simulink model "ansiBPF"  (R2018a)
settings: Solver=VariableStepAuto  StartTime=0.0  StopTime=0.001  RelTol=1e-3
undefined symbols (not defined in the file): fdesignblkfcn, G1, G10, G11, G12, G13, G14, G15, G16, G17, G18, G19, G2, G20, G21, G22, G23, G24, G25, G26, G3, G4, G5, G6, G7, G8, G9, gcbh, get, T
libraries: dspsrcs4 x1, dspxfrm3 x1, dspobslib x1
(part 8 of 8)

== system ansiBPF/Filter Bank /Filter 7/Bandpass Filter ==
  In : Inport
  Generated Filter Block : DiscreteFir  Tag=BlockMethodSubSystem  Coefficients=[-0.00513428504174898853 -0.000361211182980185862 -0.000373103186357564155 -0.000384811331785065228 -0.000396112667542441576 -0.000407118555369722311 -0.000417653688197336121 -0.000427763725028186906 -0.000437267124181367581 -0.000446249305343924966 -0.000454509424433863511 -0.000462144016945200342 -0.000468961541006500285 -0.00047510108603985809 -0.000480378661032834482 -0.000484955245458708502 -0.000488642490353076247 -0.000491641885964510974 -0.000493768806337300647 -0.000495248235932606025 -0.000495834603735094046 -0.000495723671978558081 -0.000494559737024913965 -0.000492503002177277277 -0.000489046555423059792 -0.000484334433113684567 -0.000477752667274562498 -0.000469736939490140309 -0.000459918134660938348 -0.000449820271314354311 -0.000440410655265032196 -0.000437343681880778001 -0.000415017077466513619 -0.000403028957904219749 -0.000387890543032657796 -0.000370831057829995689 -0.000352862955276029514 -0.000333297903416547386 -0.000312652166365081177 -0.000290495949674185797 -0.000267228447718805549 -0.000242500256187110872 -0.000216622507784609391 -0.000189306018353237692 -0.000160822312630247454 -0.00013090431231813814 -9.977491882814921e-05 -6.71828741737578035e-05 -3.3362190465583284e-05 1.87737953330797842e-06 3.82578750794589309e-05 7.59296875815955528e-05 0.000114590062210208948 0.000154392763453061534 0.000195060270031960137 0.000236865934738083922 0.000279648893625907338 0.000323829091085882251 0.000369138505596120121 0.000415800723553011854 0.000462889030708697757 0.000510071506735421164 0.000556666261009906545 0.000608453913411027272 0.000657171616570307086 0.000707564922296681671 0.000758656123872777834 0.000809979435514389368 0.000861877681813531566 0.000914029787083755823 0.000966573126424342326 0.00101924401116606795 0.00107213769902803134 0.00112502250686530997 0.00117793740491828791 0.00123065410311573283 0.00128320856734487278 0.00133542131582664548 0.00138735182905208717 0.00143883522759182827 0.00148991568918932895 0.00154040519539005148 0.00159031610175726043 0.00163940693647644841 0.00168764727947417928 0.00173477135550877495 0.00178082983361215483 0.00182567127317073566 0.0018695019177895505 0.00191212963348372819 0.00195362536784609393 0.00199334896058852478 0.00203113833753347474 0.00206700493227391681 0.0021029201432464506 0.00213512724940612131 0.00216618711059341461 0.00219526175881140173 0.0022220427721179898 0.00224678560238826585 0.00226918834154568681 0.00228934830816726479 0.00230704121418263746 0.00232235771406847031 0.00233510070426523435 0.00234530486231102541 0.00235276167382800173 0.00235749633401698133 0.00235933903264844667 0.00235834137161671951 0.00235436391360369047 0.00234747670652394984 0.00233755877697023988 0.00232468177547491897 0.00230868814289701641 0.00228959846568288668 0.00226721357335321659 0.00224160611906860582 0.00221267617648638086 0.00218063539614888561 0.00214536781771183446 0.00210698698475577035 0.00206506784763389392 0.00201966991007280225 0.00197100617659200792 0.00191989706014282762 0.00186440389211500507 0.00180628021157354097 0.00174486314747820904 0.00168008694999815535 0.00161223713228134309 0.00154115078309086367 0.00146698945678845746 0.00138969143960892649 0.00130944179231868717 0.0012262142007846452 0.00114015129668698623 0.00105121700108983256 0.000959543531271865027 0.00086511792793485579 0.000768083684632907249 0.000668448112385646451 0.000566380537741520483 0.000461926118994698733 0.000355279617939186323 0.000246467302056672586 0.000135638513742188267 2.27743015301716597e-05 -9.19400378440655725e-05 -0.000208443181019318563 -0.00032643762964840433 -0.000445883130048132853 -0.000566569052997391797 -0.000688684043530423361 -0.000811979045388096601 -0.000936108974577499705 -0.00106067060247101242 -0.00118658653091919348 -0.00131250527363708049 -0.00143887628290320321 -0.00156555167828120799 -0.00169215833900483942 -0.00181874382778180388 -0.0019450460938826577 -0.00207100845483666361 -0.00219634459459971607 -0.00232096893781466715 ...(+10100 chars)]  InputProcessing=Columns as channels (frame based)
  Out : Outport
  wires:
  In/1 -> Generated Filter Block/1
  Generated Filter Block/1 -> Out/1

== system ansiBPF/Filter Bank /Filter 8/Bandpass Filter ==
  In : Inport
  Generated Filter Block : DiscreteFir  Tag=BlockMethodSubSystem  Coefficients=[-0.00516622582828563971 -0.000470469850453975741 -0.000490549882434943539 -0.000510272576474730781 -0.000529259103219038157 -0.000547443950766350086 -0.000564418046489216681 -0.00058024415585958191 -0.000594695099131715976 -0.000608171258508255833 -0.000620765185585862335 -0.000633135229341045234 -0.000645123384864209996 -0.000656270670386141161 -0.000663245745322524859 -0.000659742382948630759 -0.000672197461219179414 -0.000672208555159389473 -0.000672631669906842596 -0.000670907256343796117 -0.000667146276999160993 -0.000661267229828134059 -0.00065335939409474561 -0.000643501710941031188 -0.00063162481365998651 -0.000617563186647901788 -0.000600816070578684934 -0.000581118794948503985 -0.000558593427527817425 -0.00053468284353439411 -0.000510134004286506675 -0.000478549656656596274 -0.000447614644824903367 -0.000412857540250242093 -0.000375723055969432763 -0.00033599893238356153 -0.000293788202406544338 -0.000249025996370232788 -0.000201615208860929027 -0.000151506950943869692 -9.87495026655666949e-05 -4.36860094795753565e-05 1.34369612407574807e-05 7.26848610468847772e-05 0.000134868178762570512 0.000199886430919735472 0.000265172162908887052 0.000334111893832970963 0.000404158133811660485 0.000476233265677101364 0.000549994935729505863 0.000625460031310635066 0.000702474439985669233 0.000780822993068162018 0.000860275966794977164 0.000940660153755685548 0.00102204731506121745 0.00110444048473083874 0.00118757515810453441 0.0012707203539297704 0.00135391275927980621 0.00143810528473717683 0.00152120728030154685 0.00160462552478224385 0.00168738456167015841 0.00176953439616191633 0.00185072216352515084 0.00193074754199950779 0.00200945791714424171 0.00208673054518639448 0.00216240126773788871 0.00223608320712765339 0.00230743874758019109 0.00237633712512425694 0.00244293042463733685 0.00250675957990770422 0.00256708344849166173 0.00262484203203490734 0.00267870525089187106 0.00272908657726209395 0.00277552643260705169 0.00281798471259865234 0.00285627410272580812 0.00289017519445788776 0.00291943051726411889 0.00294380971977944257 0.00296328334514732753 0.00297777781856333043 0.00298707128038297638 0.00299078449766026089 0.00298901586293517452 0.00298186417418701581 0.00296848300755047029 0.00294958359243369756 0.00292457078367636342 0.00289362169080571848 0.00285650644543801414 0.00281315901245932044 0.00276354479052459429 0.00270768948248704608 0.00264562478638331053 0.00257722682857348126 0.00250244525649638604 0.00242135194483165473 0.00233412011075075044 0.00224058548305073246 0.00214074097074218967 0.00203513220560679704 0.00192324114531232555 0.00180557593886658801 0.0016819929008185892 0.0015527735307927313 0.00141805819950537731 0.00127800228842972312 0.0011327280884166728 0.000982368917318102511 0.000827216960412459172 0.000667505170831749449 0.000503414648857781512 0.000335102309466787582 0.000162996299675745478 -1.2660062738425841e-05 -0.000191901271174567574 -0.000373994901280969884 -0.000558978901638184159 -0.000746298052439770682 -0.000935782046631534158 -0.00112709036725883258 -0.00131989501365202284 -0.00151381602642057696 -0.00170845729564908858 -0.00190353989913731245 -0.00209869229400019234 -0.00229351214145015383 -0.00248758457267906751 -0.0026806784836139381 -0.00287235159113056202 -0.00306202001003352342 -0.00324962484080369143 -0.0034345041600563949 -0.00361650257499006485 -0.00379509362215890191 -0.00396991988823447873 -0.00414058572212833327 -0.00430673836065147489 -0.00446804058740806701 -0.00462405483732230421 -0.00477444919506033079 -0.00491888801364138376 -0.00505703881496733215 -0.00518844176890496857 -0.00531284244977005271 -0.00543004618207943053 -0.00553950737716360844 -0.00564115351930098013 -0.00573448919213389967 -0.00581937587783869226 -0.00589551526925932365 -0.00596268221950041477 -0.00602063134083479553 -0.0060691213802247174 -0.00610801693280466941 -0.00613708840277420176 -0.00615616641601029156 -0.00616510247986063603 -0.00616386699945285083 -0.00615227565298735908 ...(+7453 chars)]  InputProcessing=Columns as channels (frame based)
  Out : Outport
  wires:
  In/1 -> Generated Filter Block/1
  Generated Filter Block/1 -> Out/1

== system ansiBPF/Filter Bank /Filter 9/Bandpass Filter ==
  In : Inport
  Generated Filter Block : DiscreteFir  Tag=BlockMethodSubSystem  Coefficients=[-0.00521622071402781315 -0.000584369089097545695 -0.000612771879296090602 -0.000640699051298466125 -0.000665292835330725217 -0.000688870324546760407 -0.000708508716363896209 -0.000727059670697887371 -0.000741576045727494575 -0.000755450877477878077 -0.000765042736214328715 -0.000773914092242260383 -0.000775617151377141871 -0.000774238148626573731 -0.000759486165946542287 -0.000756547480626466352 -0.000741703610879660032 -0.000718098395813007717 -0.000695336004581752903 -0.000663827113534123589 -0.000630134043701226741 -0.000589290264754247298 -0.000545020693067301693 -0.000493667568802856095 -0.000437956708558766977 -0.000375201833172760305 -0.000308630634861349964 -0.00023597805840165631 -0.000159791134180596595 -7.46626350228074206e-05 1.42459138302367117e-05 0.000106247532310519734 0.000205819808527946298 0.000308444438702868903 0.000416492755492746565 0.000528492173752373798 0.000644788285284607875 0.000764558039990328141 0.000887596020325012551 0.00101351356198251755 0.00114236442298529511 0.00127371527285175586 0.00140684251398512632 0.00154057386055048238 0.00167518735483513422 0.00181175710068573036 0.00194636947330776005 0.00208152773187451467 0.00221502332519264017 0.00234684821718133835 0.00247633777394765456 0.0026030246805159446 0.00272639380194544464 0.00284573790865105987 0.00296025010335355899 0.00306940268536068156 0.00317288257867006816 0.00327023171262956188 0.00336054675428869298 0.0034424965576385488 0.00351722374947801902 0.0035827931614132052 0.00363900327808223565 0.00368587063388151276 0.00372208516370736578 0.0037478213993065823 0.00376200941389866986 0.00376481934859222711 0.00375559242666084064 0.0037342255867455253 0.00369989107867593281 0.00365263430952227899 0.00359213757651698955 0.00351877459793821295 0.00343130799784788958 0.00333046305255326565 0.00321614897136979607 0.00308773528670458616 0.00294603356732238723 0.00279064610136103798 0.00262206286437159262 0.00244021061340714924 0.00224535109658622256 0.00203786799723648703 0.00181825761231623872 0.00158683669674391896 0.00134396269457104714 0.00109003372885849679 0.000826049807702892991 0.000552349818990468915 0.000269321237048327465 -2.15947788168796909e-05 -0.000320397711584988025 -0.00062589398971356347 -0.000937406384712054751 -0.00125398669329774507 -0.00157458689285554579 -0.00189850293296120031 -0.00222470398951584315 -0.0025521943981579461 -0.00287979354333768112 -0.00320652545528318485 -0.00353144941388871527 -0.00385344562088116207 -0.00417109498111363844 -0.00448394808417981218 -0.00479029720335497934 -0.00508928112864834824 -0.00537983088545412706 -0.00566078332931819507 -0.00593126824297946116 -0.00618997112993737841 -0.00643594014922562862 -0.00666821545715900414 -0.00688586460698052769 -0.00708792380343714265 -0.00727339131624225171 -0.0074414778910253717 -0.00759153761638956502 -0.00772241438799983401 -0.00783372644040708846 -0.00792484065501518342 -0.00799488975214572226 -0.00804360863783262769 -0.00807023543358698428 -0.00807466419979072786 -0.00805644258941918753 -0.00801525627313023729 -0.00795092600645391605 -0.0078633359681095933 -0.00775250407462602185 -0.00761840535831301378 -0.0074610561366464977 -0.00728088973544778473 -0.00707798702550464613 -0.00685255004015525825 -0.00660535141313611969 -0.00633657935795974275 -0.00604705050477750191 -0.00573718313758251469 -0.00540776196870100707 -0.00505967040739718071 -0.00469368827064281513 -0.00431075333033423009 -0.00391184817269122666 -0.00349800884290560376 -0.00307045600771758661 -0.00263012090636695469 -0.00217840569209117778 -0.00171664926755677513 -0.00124590655518394197 -0.000767673764111516214 -0.00028330063585945385 0.00020582201083028679 0.000698114955651565373 0.0011924125718660479 0.00168697372878823162 0.00218049071308427586 0.00267137229768290045 0.00315820952006252076 0.00363949892753647267 0.0041137123746689359 0.00457942419750878918 0.00503539751575623508 0.005479876506709256 0.00591170855737786077 0.00632948725870542336 0.00673192051803647717 ...(+4716 chars)]  InputProcessing=Columns as channels (frame based)
  Out : Outport
  wires:
  In/1 -> Generated Filter Block/1
  Generated Filter Block/1 -> Out/1
